simulink model "matcher_simu"  (R2024b)
settings: Solver=FixedStepDiscrete  StartTime=0.0  StopTime=N_sym  RelTol=1e-3
InitFcn:
  | %% DSPBuilder Start
  | alt_dspbuilder_update_model(bdroot)
  | %% DSPBuilder End
  | 
  | matcher_init
StartFcn:
  | %% DSPBuilder Start
  | alt_dspbuilder_hdlimport_prepare_for_simulation(bdroot)
  | %% DSPBuilder End
StopFcn:
  | matcher_analysis
undefined symbols (not defined in the file or in its folder): state
libraries: allblocks_alteradspbuilder2 x38, dspsrcs4 x2
settings Model: Creator=vboxuser  LastModifiedBy=piotr
settings SolverCC: AlgebraicLoopSolver=TrustRegion
settings DataIOCC: SaveFormat=Array
settings DebuggingCC: UnconnectedInputMsg=warning  UnconnectedOutputMsg=warning  UnconnectedLineMsg=warning
settings ModelReferenceCC: EnableRefExpFcnMdlSchedulingChecks=on
settings RTWCC: GPUComputeCapability=3.5

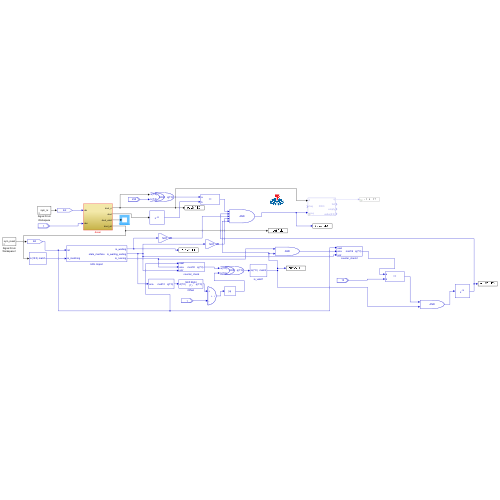
[thumbnail: Simulink's stored preview of the top-level diagram]
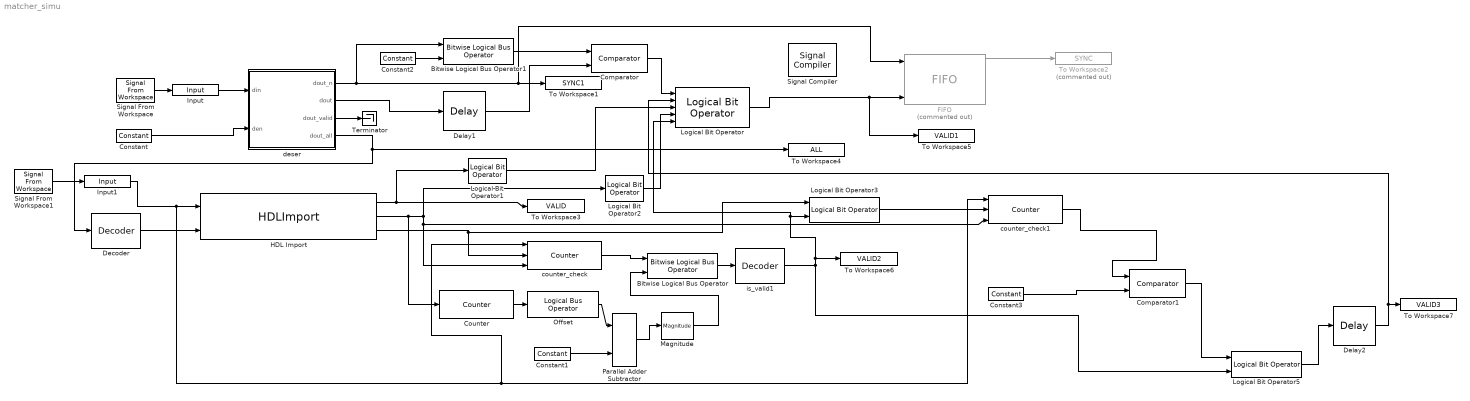
== system matcher_simu ==
  Bitwise Logical Bus Operator : allblocks_alteradspbuilder2/Bitwise Logical Bus Operator  BusType=Unsigned Integer  bwl=8  bwr=0  LogicalOperator=XOR  pipeline_display=0
  Bitwise Logical Bus Operator1 : allblocks_alteradspbuilder2/Bitwise Logical Bus Operator  BusType=Unsigned Integer  bwl=8  bwr=0  LogicalOperator=XOR  pipeline_display=0
  Comparator : allblocks_alteradspbuilder2/Comparator  direction=a == b  pipeline_display=0  allowFloatingPointOverride=on  logOutputs=off  logFile=D:\programowanie\studia\ids\system2\tb_matcher_simu\matcher%5Fsimu_Comparator.fixedpointlog
  Comparator1 : allblocks_alteradspbuilder2/Comparator  direction=a == b  pipeline_display=0  allowFloatingPointOverride=on  logOutputs=off  logFile=D:\programowanie\studia\ids\system2\tb_matcher_simu\matcher%5Fsimu_Comparator1.fixedpointlog
  Constant : allblocks_alteradspbuilder2/Constant  mask_cst=1  BusType=Single Bit  bwl=8  bwr=0  roundMode=Truncate  satMode=Wrap  SpecifyClock=off  allowFloatingPointOverride=on  logOutputs=off  logFile=D:\programowanie\studia\ids\system2\tb_matcher_simu\matcher%5Fsimu_Constant.fixedpointlog
  Constant1 : allblocks_alteradspbuilder2/Constant  mask_cst=1  BusType=Unsigned Integer  bwl=8  bwr=0  roundMode=Truncate  satMode=Wrap  SpecifyClock=off  allowFloatingPointOverride=on  logOutputs=off  logFile=D:\programowanie\studia\ids\system2\tb_matcher_simu\matcher%5Fsimu_Constant1.fixedpointlog
  Constant2 : allblocks_alteradspbuilder2/Constant  mask_cst=0b11111111  BusType=Unsigned Integer  bwl=8  bwr=0  roundMode=Truncate  satMode=Wrap  SpecifyClock=off  allowFloatingPointOverride=on  logOutputs=off  logFile=D:\programowanie\studia\ids\system2\tb_matcher_simu\matcher%5Fsimu_Constant2.fixedpointlog
  Constant3 : allblocks_alteradspbuilder2/Constant  mask_cst=15  BusType=Unsigned Integer  bwl=8  bwr=0  roundMode=Truncate  satMode=Saturate  SpecifyClock=off  allowFloatingPointOverride=on  logOutputs=off  logFile=D:\programowanie\studia\ids\system2\tb_matcher_simu\matcher%5Fsimu_Constant3.fixedpointlog
  Counter : allblocks_alteradspbuilder2/Counter  BusType=Unsigned Integer  bwl=8  bwr=0  use_modulo=on  modulo=10  SpecifyClock=off  direction=Increment  use_sload=off  use_sset=off  svalue=1  use_clk_ena=off  use_ena=on  use_sclr=off  pipeline_display=1
  Decoder : allblocks_alteradspbuilder2/Decoder  BusType=Unsigned Integer  bwl=16  bwr=2  registered=on  pipeline_display=1  value=22182
  Delay1 : allblocks_alteradspbuilder2/Delay  pipeline=10  pipeline_display=10  ClockPhase=1  use_ena=off  use_sclr=off  allowFloatingPointOverride=on  logOutputs=off  logFile=D:\programowanie\studia\ids\system2\tb_matcher_simu\matcher%5Fsimu_Delay1.fixedpointlog  use_init=off  reset_value=1
  Delay2 : allblocks_alteradspbuilder2/Delay  pipeline=10  pipeline_display=10  ClockPhase=1  use_ena=off  use_sclr=off  allowFloatingPointOverride=on  logOutputs=off  logFile=D:\programowanie\studia\ids\system2\tb_matcher_simu\matcher%5Fsimu_Delay2.fixedpointlog  use_init=off  reset_value=1
  FIFO : allblocks_alteradspbuilder2/FIFO  Commented=on  numwords=64  BusType=Signed Integer  bwl=8  bwr=0  ram_type=AUTO  use_sclr=off  use_les_only=off  showahead_mode=on  allowFloatingPointOverride=on  logOutputs=off  logFile=D:\programowanie\studia\ids\system2\tb_matcher_simu\matcher%5Fsimu_FIFO%3A%3Aq.fixedpointlog,D:\programowanie\studia\ids\system2\tb_matcher_simu\matcher%5Fsimu_FIFO%3A%3Afull.fixedpointlog,D:\programowanie\studia\ids\system2\tb_matcher_simu\matcher%5Fsimu_FIFO%3A%3Aempty.fixedpointlog,D:\programowanie\studia\ids\system2\tb_matcher_simu\matcher%5Fsimu_FIFO%3A%3Ausedw.fixedpointlog,
  HDL Import : allblocks_alteradspbuilder2/HDLImport  entityName=state_machine_import  inNames=rst is_matching  inBwls=1 1  inBwrs="0  0"  inTypes=b b  inDelayed="0  0"  outNames=is_waiting is_waiting_ending is_running  outBwls=1 1 1  outBwrs="0  0  0"  outTypes=b b b  xmlmapfile=D:\pliki-programow\intel\18.1\quartus\dsp_builder\lib\SimgenCMap.xml  vofile=DSPBuilder_matcher_simu_import\state_machine.vo  src_file=state.v;  TopLevelName=state_machine  UseQPF=0  n_input_port=2  n_output_port=3  array_clocks=clk  use_systemC_model=off  is_megacore=off  use_dynamic_feedthrough_data=off  use_alphabetical_port_ordering=off  allowFloatingPointOverride=off  id=0  id_is_set=off  UseModelSimBasedFlow=off
  Input : allblocks_alteradspbuilder2/Input  iofile=D:\programowanie\studia\ids\system2\tb_matcher_simu\matcher%5Fsimu_Input.salt  BusType=Single Bit  bwl=8  bwr=0  SpecifyClock=off  PORTTYPE=Input  externalType=Inferred  allowFloatingPointOverride=on  logOutputs=off
  Input1 : allblocks_alteradspbuilder2/Input  iofile=D:\programowanie\studia\ids\system2\tb_matcher_simu\matcher%5Fsimu_Input1.salt  BusType=Single Bit  bwl=8  bwr=0  SpecifyClock=off  PORTTYPE=Input  externalType=Inferred  allowFloatingPointOverride=on  logOutputs=off
  Logical Bit Operator : allblocks_alteradspbuilder2/Logical Bit Operator  LogicalOperator=AND  user_inputs=5  pipeline_display=0
  Logical Bit Operator1 : allblocks_alteradspbuilder2/Logical Bit Operator  LogicalOperator=NOT  user_inputs=2  pipeline_display=0
  Logical Bit Operator2 : allblocks_alteradspbuilder2/Logical Bit Operator  LogicalOperator=NOT  user_inputs=2  pipeline_display=0
  Logical Bit Operator3 : allblocks_alteradspbuilder2/Logical Bit Operator  LogicalOperator=AND  user_inputs=2  pipeline_display=0
  Logical Bit Operator5 : allblocks_alteradspbuilder2/Logical Bit Operator  LogicalOperator=AND  user_inputs=2  pipeline_display=0
  Magnitude : allblocks_alteradspbuilder2/Magnitude  pipeline_display=0
  Offset : allblocks_alteradspbuilder2/Logical Bus Operator  BusType=Unsigned Integer  bwl=8  bwr=0  LogicalOp_text=Shift Right  mask_value_num=-5  shift_amount=1  force_sign_ext=on  pipeline_display=0
  Parallel Adder Subtractor : allblocks_alteradspbuilder2/Parallel Adder Subtractor  number_of_inputs=2  direction=+-  use_pipeline=on  pipeline_display=1  phase_selection=1  use_ena=off  use_aclr=off  allowFloatingPointOverride=on  logOutputs=off  logFile=D:\programowanie\studia\ids\system2\tb_matcher_simu\matcher%5Fsimu_Parallel+Adder+Subtractor.fixedpointlog
  Signal Compiler : allblocks_alteradspbuilder2/Signal Compiler  DeviceFamily=Cyclone IV E  DeviceName=AUTO  DisableEarlyHDLGeneration=off  EnableSignalTap=off  SignalTapDepth=128  UseBoardBlock=off  StpUseDefaultClock=on  StpClock=Clock  ExportDir=D:\pliki-programow\intel\18.1\quartus\dsp_builder  MAX10_ProgrammingMode=Internal Flash (SDM) Single Boot
  Signal From Workspace : dspsrcs4/Signal From Workspace  X=sym_rx  Ts=1  nsamps=1  OutputAfterFinalValue=Setting to zero  ignoreOrWarnInputAndFrameLengths=off  OutputFrames=off
  Signal From Workspace1 : dspsrcs4/Signal From Workspace  X=sym_reset  Ts=1  nsamps=1  OutputAfterFinalValue=Setting to zero  ignoreOrWarnInputAndFrameLengths=off  OutputFrames=off
  Terminator : Terminator
  To Workspace1 : ToWorkspace  VariableName=SYNC1  SampleTime=-1
      settings: Save2DSignal=2-D array (concatenate along first dimension)
  To Workspace2 : ToWorkspace  Commented=on  VariableName=SYNC  SampleTime=-1
      settings: Save2DSignal=2-D array (concatenate along first dimension)
  To Workspace3 : ToWorkspace  VariableName=VALID  SampleTime=-1
      settings: Save2DSignal=2-D array (concatenate along first dimension)
  To Workspace4 : ToWorkspace  VariableName=ALL  SampleTime=-1
      settings: Save2DSignal=2-D array (concatenate along first dimension)
  To Workspace5 : ToWorkspace  VariableName=VALID1  SampleTime=-1
      settings: Save2DSignal=2-D array (concatenate along first dimension)
  To Workspace6 : ToWorkspace  VariableName=VALID2  SampleTime=-1
      settings: Save2DSignal=2-D array (concatenate along first dimension)
  To Workspace7 : ToWorkspace  VariableName=VALID3  SampleTime=-1
      settings: Save2DSignal=2-D array (concatenate along first dimension)
  counter_check : allblocks_alteradspbuilder2/Counter  BusType=Unsigned Integer  bwl=8  bwr=0  use_modulo=on  modulo=10  SpecifyClock=off  direction=Increment  use_sload=off  use_sset=on  svalue=1  use_clk_ena=off  use_ena=on  use_sclr=on  pipeline_display=1
  counter_check1 : allblocks_alteradspbuilder2/Counter  BusType=Unsigned Integer  bwl=8  bwr=0  use_modulo=on  modulo=16  SpecifyClock=off  direction=Increment  use_sload=off  use_sset=on  svalue=1  use_clk_ena=off  use_ena=on  use_sclr=on  pipeline_display=1
  deser : Subsystem
  is_valid1 : allblocks_alteradspbuilder2/Decoder  BusType=Unsigned Integer  bwl=8  bwr=2  registered=on  pipeline_display=1  value=0
  wires:
  Signal From Workspace/1 -> Input/1
  Input/1 -> deser/1(din)
  deser/1(dout_n) -> FIFO/1, To Workspace1/1, Bitwise Logical Bus Operator1/1
  Constant/1 -> deser/2(den)
  Signal From Workspace1/1 -> Input1/1
  deser/4(dout_all) -> To Workspace4/1, Decoder/1
  Decoder/1 -> HDL Import/2
  HDL Import/2 -> counter_check/3, counter_check1/3, Logical Bit Operator2/1, Counter/1
  Counter/1 -> Offset/1
  HDL Import/3 -> counter_check/2, Logical Bit Operator3/1
  counter_check/1 -> Bitwise Logical Bus Operator/1
  Constant2/1 -> Bitwise Logical Bus Operator1/2
  Bitwise Logical Bus Operator1/1 -> Comparator/1
  Comparator/1 -> Logical Bit Operator/1
  deser/2(dout) -> Delay1/1
  Delay1/1 -> Comparator/2
  Logical Bit Operator/1 -> To Workspace5/1, FIFO/3
  HDL Import/1 -> To Workspace3/1, Logical Bit Operator1/1
  Logical Bit Operator1/1 -> Logical Bit Operator/3
  Input1/1 -> counter_check/1, counter_check1/1, HDL Import/1
  Logical Bit Operator2/1 -> Logical Bit Operator/4
  Constant1/1 -> Parallel Adder Subtractor/2
  Offset/1 -> Parallel Adder Subtractor/1
  Parallel Adder Subtractor/1 -> Magnitude/1
  Bitwise Logical Bus Operator/1 -> is_valid1/1
  is_valid1/1 -> Logical Bit Operator5/2, Logical Bit Operator3/2, Logical Bit Operator/5, To Workspace6/1
  Magnitude/1 -> Bitwise Logical Bus Operator/2
  Comparator1/1 -> Logical Bit Operator5/1
  Constant3/1 -> Comparator1/2
  Logical Bit Operator3/1 -> counter_check1/2
  counter_check1/1 -> Comparator1/1
  Logical Bit Operator5/1 -> Delay2/1
  Delay2/1 -> To Workspace7/1, Logical Bit Operator/2
  FIFO/1 -> To Workspace2/1
  deser/3(dout_valid) -> Terminator/1

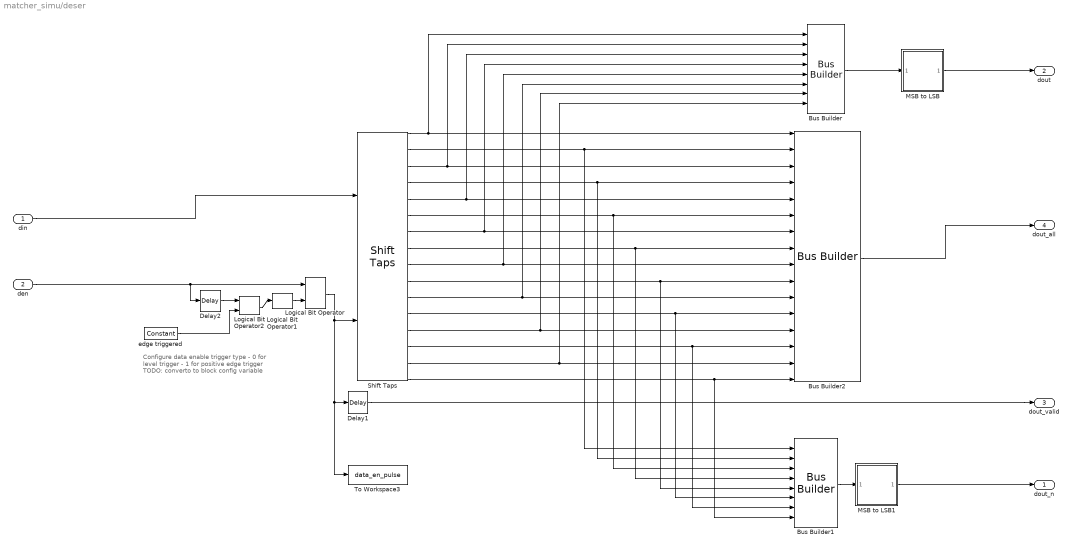
== system matcher_simu/deser ==
  note: Configure data enable trigger type
      |  - 0 for level trigger
      |  - 1 for positive edge trigger
      |
      | TODO: converto to block config variable
  din : Inport
  den : Inport  Port=2
  Bus Builder : allblocks_alteradspbuilder2/Bus Builder  BusType=Unsigned Integer  bwl=8  bwr=1  pipeline_display=0
  Bus Builder1 : allblocks_alteradspbuilder2/Bus Builder  BusType=Unsigned Integer  bwl=8  bwr=1  pipeline_display=0
  Bus Builder2 : allblocks_alteradspbuilder2/Bus Builder  BusType=Unsigned Integer  bwl=16  bwr=1  pipeline_display=0
  Delay1 : allblocks_alteradspbuilder2/Delay  pipeline=1  pipeline_display=1  ClockPhase=1  use_ena=off  use_sclr=off  allowFloatingPointOverride=on  logOutputs=off  logFile=D:\programowanie\studia\ids\system2\tb_matcher_simu\matcher%5Fsimu_deser_Delay1.fixedpointlog  use_init=off  reset_value=1
  Delay2 : allblocks_alteradspbuilder2/Delay  pipeline=1  pipeline_display=1  ClockPhase=1  use_ena=off  use_sclr=off  allowFloatingPointOverride=on  logOutputs=off  logFile=D:\programowanie\studia\ids\system2\tb_matcher_simu\matcher%5Fsimu_deser_Delay2.fixedpointlog  use_init=off  reset_value=1
  Logical Bit Operator : allblocks_alteradspbuilder2/Logical Bit Operator  LogicalOperator=AND  user_inputs=2  pipeline_display=0
  Logical Bit Operator1 : allblocks_alteradspbuilder2/Logical Bit Operator  LogicalOperator=NOT  user_inputs=2  pipeline_display=0
  Logical Bit Operator2 : allblocks_alteradspbuilder2/Logical Bit Operator  LogicalOperator=AND  user_inputs=2  pipeline_display=0
  MSB to LSB : Subsystem  ReferencedSubsystem=MSB_to_LSB
  MSB to LSB1 : Subsystem  ReferencedSubsystem=MSB_to_LSB
  Shift Taps : allblocks_alteradspbuilder2/Shift Taps  number_of_taps=16  tap_distance=10  use_shiftout=off  use_ena=on  use_sclr=off  use_dedicated_circuitry=on  ram_type=AUTO  allowFloatingPointOverride=on  logOutputs=off  logFile=D:\programowanie\studia\ids\system2\tb_matcher_simu\matcher%5Fsimu_deser_Shift+Taps%3A%3At.fixedpointlog,D:\programowanie\studia\ids\system2\tb_matcher_simu\matcher%5Fsimu_deser_Shift+Taps%3A%3At.fixedpointlog,D:\programowanie\studia\ids\system2\tb_matcher_simu\matcher%5Fsimu_deser_Shift+Taps%3A%3At.fixedpointlog,D:\programowanie\studia\ids\system2\tb_matcher_simu\matcher%5Fsimu_deser_Shift+Taps%3A%3At.fixedpointlog,D:\programowanie\studia\ids\system2\tb_matcher_simu\matcher%5Fsimu_deser_Shift+Taps%3A%3At.fixedpointlog,D:\programowanie\studia\ids\system2\tb_matcher_simu\matcher%5Fsimu_deser_Shift+Taps%3A%3At.fixedpointlog,D:\programowanie\studia\ids\system2\tb_matcher_simu\matcher%5Fsimu_deser_Shift+Taps%3A%3At.fixedpointlog,D:\programowanie\studia\ids\system2\tb_matcher_simu\matcher%5Fsimu_deser_Shift+Taps%3A%3At.fixedpointlog,D:\programowanie\studia\ids\system2\tb_matcher_simu\matcher%5Fsimu_deser_Shift+Taps%3A%3At.fixedpointlog,D:\programowanie\studia\ids\system2\tb_matcher_simu\matcher%5Fsimu_deser_Shift+Taps%3A%3At.fixedpointlog,D:\programowanie\studia\ids\system2\tb_matcher_simu\matcher%5Fsimu_deser_Shift+Taps%3A%3At.fixedpointlog,D:\programowanie\studia\ids\system2\tb_matcher_simu\matcher%5Fsimu_deser_Shift+Taps%3A%3At.fixedpointlog,D:\programowanie\studia\ids\system2\tb_matcher_simu\matcher%5Fsimu_deser_Shift+Taps%3A%3At.fixedpointlog,D:\programowanie\studia\ids\system2\tb_matcher_simu\matcher%5Fsimu_deser_Shift+Taps%3A%3At.fixedpointlog,D:\programowanie\studia\ids\system2\tb_matcher_simu\matcher%5Fsimu_deser_Shift+Taps%3A%3At.fixedpointlog,D:\programowanie\studia\ids\system2\tb_matcher_simu\matcher%5Fsimu_deser_Shift+Taps%3A%3At.fixedpointlog,
  To Workspace3 : ToWorkspace  VariableName=data_en_pulse  SampleTime=-1
      settings: Save2DSignal=2-D array (concatenate along first dimension)
  edge triggered : allblocks_alteradspbuilder2/Constant  mask_cst=0  BusType=Single Bit  bwl=8  bwr=0  roundMode=Truncate  satMode=Wrap  SpecifyClock=off  allowFloatingPointOverride=on  logOutputs=off  logFile=D:\programowanie\studia\ids\system2\tb_matcher_simu\matcher%5Fsimu_deser_edge+triggered.fixedpointlog
  dout_n : Outport
  dout : Outport  Port=2
  dout_valid : Outport  Port=3
  dout_all : Outport  Port=4
  wires:
  din/1 -> Shift Taps/1
  MSB to LSB/1 -> dout/1
  edge triggered/1 -> Logical Bit Operator2/2
  MSB to LSB1/1 -> dout_n/1
  Shift Taps/8 -> Bus Builder1/4, Bus Builder2/8
  den/1 -> Logical Bit Operator/1, Delay2/1
  Logical Bit Operator1/1 -> Logical Bit Operator/2
  Shift Taps/12 -> Bus Builder1/6, Bus Builder2/12
  Shift Taps/7 -> Bus Builder/4, Bus Builder2/7
  Logical Bit Operator/1 -> Shift Taps/2, To Workspace3/1, Delay1/1
  Shift Taps/10 -> Bus Builder1/5, Bus Builder2/10
  Shift Taps/14 -> Bus Builder1/7, Bus Builder2/14
  Delay1/1 -> dout_valid/1
  Shift Taps/1 -> Bus Builder/1, Bus Builder2/1
  Bus Builder2/1 -> dout_all/1
  Logical Bit Operator2/1 -> Logical Bit Operator1/1
  Shift Taps/13 -> Bus Builder/7, Bus Builder2/13
  Shift Taps/9 -> Bus Builder/5, Bus Builder2/9
  Shift Taps/15 -> Bus Builder/8, Bus Builder2/15
  Bus Builder1/1 -> MSB to LSB1/1
  Shift Taps/11 -> Bus Builder/6, Bus Builder2/11
  Shift Taps/16 -> Bus Builder2/16, Bus Builder1/8
  Shift Taps/4 -> Bus Builder1/2, Bus Builder2/4
  Delay2/1 -> Logical Bit Operator2/1
  Shift Taps/3 -> Bus Builder/2, Bus Builder2/3
  Shift Taps/2 -> Bus Builder1/1, Bus Builder2/2
  Bus Builder/1 -> MSB to LSB/1
  Shift Taps/5 -> Bus Builder/3, Bus Builder2/5
  Shift Taps/6 -> Bus Builder1/3, Bus Builder2/6
